simulink model "Q3_simulink"  (R2024b)
settings: Solver=VariableStepAuto  StartTime=0.0  StopTime=10.0  RelTol=1e-3
settings Model: Creator=Sagar  LastModifiedBy=Sagar

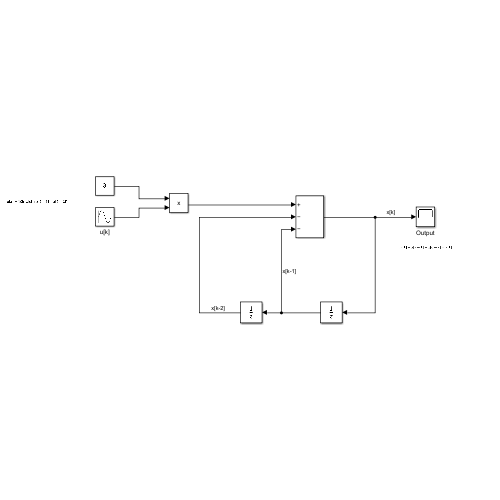
[thumbnail: Simulink's stored preview of the top-level diagram]
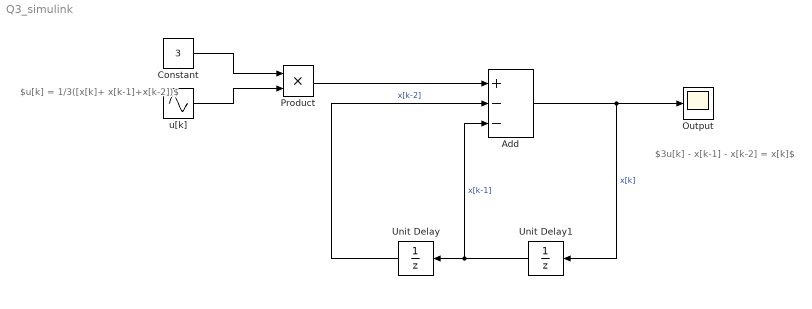
== system Q3_simulink ==
  note: $u[k] = 1/3([x[k]+ x[k-1]+x[k-2])$
  note: $3u[k] - x[k-1] - x[k-2] = x[k]$
  Add : Sum  Inputs=+--
  Constant : Constant  Value=3
  Output : Scope
  Product : Product
  Unit Delay : UnitDelay  SampleTime=-1  HasFrameUpgradeWarning=on
  Unit Delay1 : UnitDelay  SampleTime=-1  HasFrameUpgradeWarning=on
  u[k] : Sin  SampleTime=0
  wires:
  u[k]/1 -> Product/2
  Unit Delay1/1 -> Add/3, Unit Delay/1  "x[k-1]"
  Unit Delay/1 -> Add/2  "x[k-2]"
  Add/1 -> Output/1, Unit Delay1/1  "x[k]"
  Constant/1 -> Product/1
  Product/1 -> Add/1
